simulink model "DKDC"  (R2013b)
settings: Solver=ode5  StartTime=0.0  StopTime=inf  FixedStep=0.01  RelTol=1e-3
undefined symbols (not defined in the file or in its folder): National_Instruments, PCI
libraries: rtwinlib x4, simulink x1
settings Model: SimulationMode=external  Creator=Administrator  LastModifiedBy=Administrator
settings HardwareCC: ProdIntDivRoundTo=Zero  ProdEndianess=LittleEndian  ProdHWDeviceType=Generic->32-bit x86 compatible
settings RTWCC: SystemTargetFile=rtwin.tlc  TemplateMakefile=rtwin.tmf  Description=Real-Time Windows Target  ProcessScript=rtwin_make_rtw_hook  RTWCompilerOptimization=On
settings CodeAppCC: MaxIdLength=95
settings RTWinTargetCC: TargetLibSuffix=_rtwin.lib  TargetPreCompLibLocation=C:\Program Files\MATLAB\R2013b\toolbox\rtw\targets\rtwin\lib\win64  CodeReplacementLibrary=ANSI_C  RTWinDir=C:/PROGRA~1/MATLAB/R2013b/toolbox/rtw/targets/rtwin  TargetArch=win64

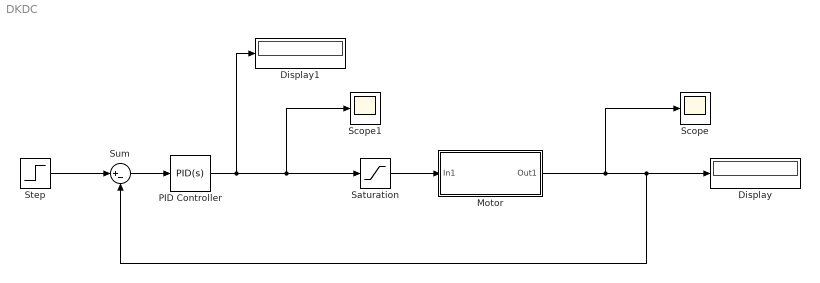
== system DKDC ==
  Display : Display
  Display1 : Display
  "Motor " : Subsystem
  PID Controller : simulink/Continuous/PID Controller  Controller=PID  TimeDomain=Continuous-time  SampleTime=1  IntegratorMethod=Forward Euler  FilterMethod=Forward Euler  Form=Parallel  P=0.0052  I=0.05  D=0  N=100  InitialConditionSource=internal  InitialConditionForIntegrator=0  InitialConditionForFilter=0  ExternalReset=none  LimitOutput=off  UpperSaturationLimit=inf  LowerSaturationLimit=-inf  LinearizeAsGain=on  AntiWindupMode=none  Kb=1  TrackingMode=off  Kt=1  PParamMin=[]  PParamMax=[]  IParamMin=[]  IParamMax=[]  DParamMin=[]  DParamMax=[]  NParamMin=[]  NParamMax=[]  KbParamMin=[]  KbParamMax=[]  KtParamMin=[]  KtParamMax=[]  POutMin=[]  POutMax=[]  IOutMin=[]  IOutMax=[]  DOutMin=[]  DOutMax=[]  NOutMin=[]  NOutMax=[]  KbOutMin=[]  KbOutMax=[]  KtOutMin=[]  KtOutMax=[]  IntegratorOutMin=[]  IntegratorOutMax=[]  FilterOutMin=[]  FilterOutMax=[]  SumOutMin=[]  SumOutMax=[]  SumI1OutMin=[]  SumI1OutMax=[]  SumI2OutMin=[]  SumI2OutMax=[]  SumI3OutMin=[]  SumI3OutMax=[]  SumDOutMin=[]  SumDOutMax=[]  SaturationOutMin=[]  SaturationOutMax=[]  IntegratorContinuousStateAttributes=''  IntegratorStateMustResolveToSignalObject=off  IntegratorRTWStateStorageClass=Auto  FilterContinuousStateAttributes=''  FilterStateMustResolveToSignalObject=off  FilterRTWStateStorageClass=Auto
  Saturation : Saturate  UpperLimit=20  LowerLimit=-20
  Scope : Scope
  Scope1 : Scope
      settings: YMin=1400  YMax=2350
  Step : Step  Time=0  After=1200  SampleTime=0
  Sum : Sum  Inputs=|+-
  wires:
  Saturation/1 -> "Motor "/1(In1)
  Step/1 -> Sum/1
  Sum/1 -> PID Controller/1
  PID Controller/1 -> Display1/1, Scope1/1, Saturation/1
  "Motor "/1(Out1) -> Sum/2, Display/1, Scope/1

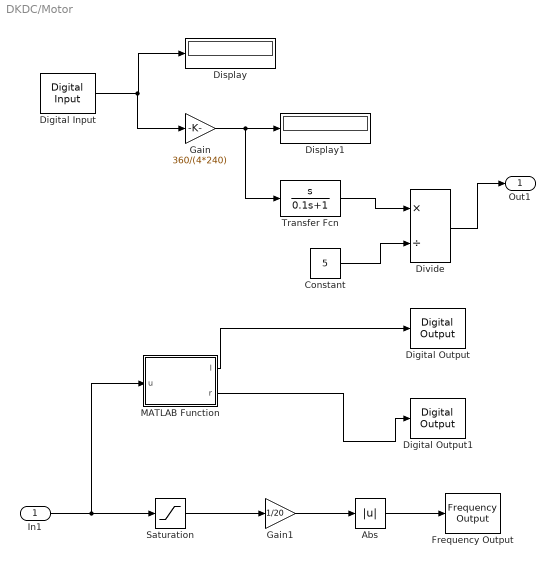
== system DKDC/Motor  ==
  In1 : Inport
  Abs : Abs
  Constant : Constant  Value=5
  Digital Input : rtwinlib/Digital Input  SampleTime=0.01  MaxMissedTicks=10  ShowMissedTicks=off  YieldWhenWaiting=off  DrvName=National_Instruments/PCI-6221  DrvAddress=4294967295  DrvOptions=[0 15 61600 2 3]  Channels=1  BitMode=1  DataType=1
      settings: AttributesFormatString=National Instruments\nPCI-6221 [auto]
  Digital Output : rtwinlib/Digital Output  SampleTime=0.01  MaxMissedTicks=10  ShowMissedTicks=off  YieldWhenWaiting=off  DrvName=National_Instruments/PCI-6221  DrvAddress=4294967295  DrvOptions=[0 15 61600 2 3]  Channels=3  BitMode=1  InitialValue=[]  FinalValue=[]
      settings: AttributesFormatString=National Instruments\nPCI-6221 [auto]
  Digital Output1 : rtwinlib/Digital Output  SampleTime=0.01  MaxMissedTicks=10  ShowMissedTicks=off  YieldWhenWaiting=off  DrvName=National_Instruments/PCI-6221  DrvAddress=4294967295  DrvOptions=[0 15 61600 2 3]  Channels=4  BitMode=1  InitialValue=[]  FinalValue=[]
      settings: AttributesFormatString=National Instruments\nPCI-6221 [auto]
  Display : Display
  Display1 : Display
  Divide : Product  Inputs=*/
  Frequency Output : rtwinlib/Frequency Output  SampleTime=0.01  MaxMissedTicks=10  ShowMissedTicks=off  YieldWhenWaiting=off  DrvName=National_Instruments/PCI-6221  DrvAddress=4294967295  DrvOptions=[0 15 61600 2 3]  Channels=2  FrequencySource=1  Frequency=1200  FrequencyFinalValue=[]  DutySource=2  Duty=0  DutyFinalValue=0
      settings: AttributesFormatString=National Instruments\nPCI-6221 [auto]
  Gain : Gain  Gain=360/(4*240)
  Gain1 : Gain  Gain=1/20
  MATLAB Function : MATLAB Function  TreatAsAtomicUnit=on
  Saturation : Saturate  UpperLimit=20  LowerLimit=-20
  Transfer Fcn : TransferFcn  Numerator=[1 0]  Denominator=[0.1 1]
  Out1 : Outport
  wires:
  Digital Input/1 -> Gain/1, Display/1
  Gain/1 -> Transfer Fcn/1, Display1/1
  Transfer Fcn/1 -> Divide/1
  Constant/1 -> Divide/2
  Divide/1 -> Out1/1
  In1/1 -> MATLAB Function/1(u), Saturation/1
  Saturation/1 -> Gain1/1
  Gain1/1 -> Abs/1
  Abs/1 -> Frequency Output/1
  MATLAB Function/1(l) -> Digital Output/1
  MATLAB Function/2(r) -> Digital Output1/1

== matlab function DKDC/Motor /MATLAB Function ==
  data: u input; l output; r output
function [l,r] = fcn(u)
if u>0
    l=0;
    r=1;
elseif u<0
    l=1;
    r=0;
else
    l=0;
    r=0;
end
